simulink model "LPF"  (Simulink 7.2)
settings: Solver=ode45  StartTime=0.0  StopTime=10.0  RelTol=1e-3
undefined symbols (not defined in the file): DiscIntNeverNeededParam
settings Model: Creator=E183308  LastModifiedBy=E183308

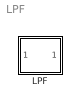
== system LPF ==
  LPF : Subsystem

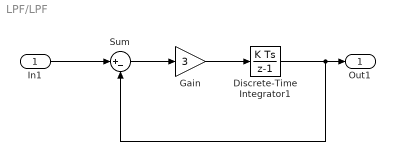
== system LPF/LPF ==
  In1 : Inport
  Discrete-Time Integrator1 : DiscreteIntegrator  SampleTime=-1  OutDataType=sfix(16)  OutScaling=2^0  ICPrevOutput=DiscIntNeverNeededParam  ICPrevScaledInput=DiscIntNeverNeededParam
  Gain : Gain  Gain=3  ParameterDataType=sfix(16)  ParameterScaling=2^0  OutDataType=sfix(16)  OutScaling=2^0
  Sum : Sum  Inputs=|+-  OutDataType=sfix(16)  OutScaling=2^0
  Out1 : Outport
  wires:
  Discrete-Time Integrator1/1 -> Out1/1, Sum/2
  In1/1 -> Sum/1
  Sum/1 -> Gain/1
  Gain/1 -> Discrete-Time Integrator1/1
